simulink model "Q44444"  (R2016b)
settings: Solver=VariableStepAuto  StartTime=0.0  StopTime=100  RelTol=1e-3
values from neighbouring files (symbols this model uses):
  a0_const = 20    [Question_4.m]
  alpha = 0.3    [Question_4.m]
  p = 1000*eye(est_param)    [Question_4.m]
  t0 = B_prim_m    [Question_4.m]
  wn = sigma/zeta    [Question_4.m]
  zeta = ((log(Mp)^2)/(pi^2+log(Mp)^2))^0.5    [Question_4.m]
libraries: cstextras x2
settings Model: Creator=vaio  LastModifiedBy=user

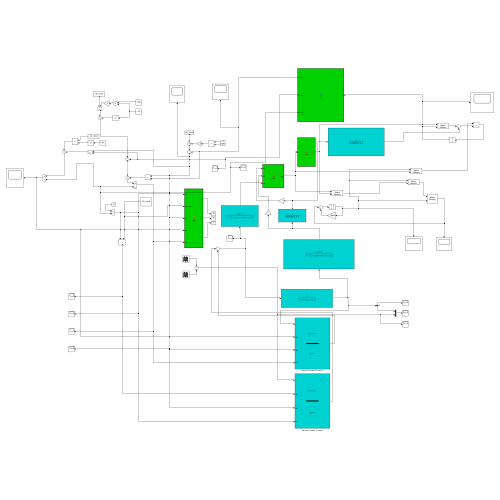
[thumbnail: Simulink's stored preview of the top-level diagram]
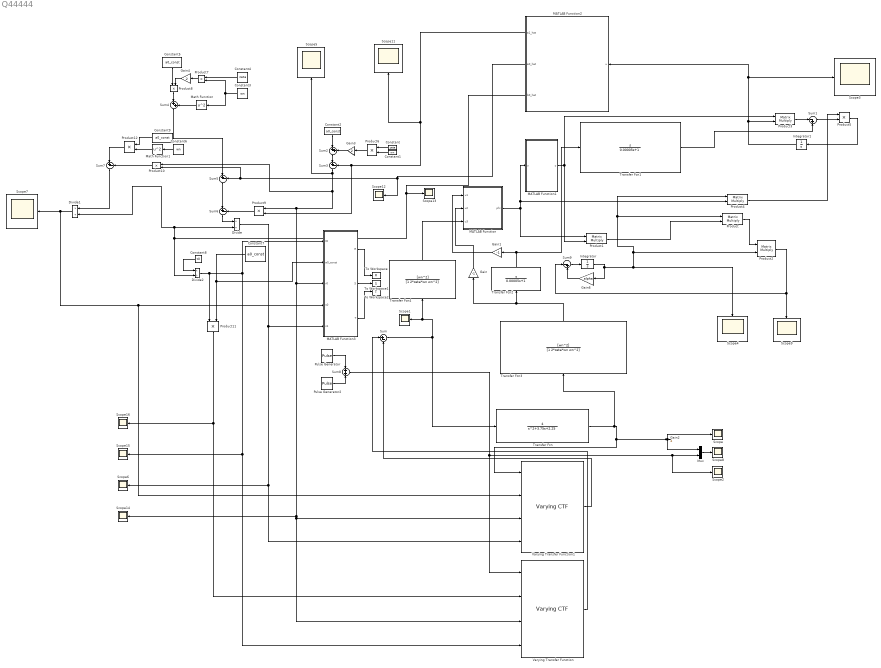
== system Q44444 ==
  Constant : Constant  Value=zeta
  Constant1 : Constant  Value=wn
  Constant{2,5,7,9} (4 alike) : Constant  Value=a0_const
  Constant3 : Constant  Value=wn
  Constant4 : Constant  Value=zeta
  Constant6 : Constant  Value=wn
  Constant8 : Constant  Value=t0
  Divide : Product  Inputs=*/
  Divide1 : Product  Inputs=*/
  Divide2 : Product  Inputs=*/
  Gain : Gain  Gain=-1
  Gain1 : Gain  Gain=-1
  Gain2 : Gain  Gain=4
  Gain3 : Gain  Gain=2
  Gain4 : Gain  Gain=2
  Gain6 : Gain  Gain=alpha
  Integrator : Integrator  InitialCondition=p  LimitOutput=on
  Integrator1 : Integrator  InitialCondition=[0.1;0.01;0.5]
  MATLAB Function : MATLAB Function  TreatAsAtomicUnit=on
  MATLAB Function1 : MATLAB Function  TreatAsAtomicUnit=on
  MATLAB Function2 : MATLAB Function  TreatAsAtomicUnit=on
  MATLAB Function3 : MATLAB Function  TreatAsAtomicUnit=on
  Math Function : Math  Operator=square  SaturateOnIntegerOverflow=on
  Math Function1 : Math  Operator=square  SaturateOnIntegerOverflow=on
  Mux : Mux  Inputs=2
  Product{,1..4} (5 alike) : Product  Multiplication=Matrix(*)
  Product{5..12} (8 alike) : Product
  Pulse Generator : DiscretePulseGenerator  PulseType=Time based  Amplitude=2  Period=50  PulseWidth=50
  Pulse Generator2 : DiscretePulseGenerator  PulseType=Time based  Amplitude=-2  Period=50  PulseWidth=50  PhaseDelay=25
  Scope{,1..9,11..16} (16 alike) : Scope
  Sum{,3,5..7} (5 alike) : Sum  Inputs=|+-
  Sum1 : Sum  Inputs=|-+
  Sum2 : Sum  Inputs=|++
  Sum4 : Sum  Inputs=|++
  Sum8 : Sum
  Sum9 : Sum  Inputs=|-+
  To Workspace : ToWorkspace  VariableName=R  SampleTime=-1
  To Workspace1 : ToWorkspace  VariableName=S  SampleTime=-1
  To Workspace2 : ToWorkspace  VariableName=T  SampleTime=-1
  Transfer Fcn : TransferFcn  Numerator=[4]  Denominator=[1 3.75 2.25]
  Transfer Fcn1 : TransferFcn  Numerator=[1 0]  Denominator=[0.00005 1]
  Transfer Fcn2 : TransferFcn  Numerator=[1 0]  Denominator=[0.00005 1]
  Transfer Fcn3 : TransferFcn  Numerator=[wn^2]  Denominator=[1 2*zeta*wn wn^2]
  Transfer Fcn4 : TransferFcn  Numerator=[wn^2]  Denominator=[1 2*zeta*wn wn^2]
  Varying Transfer Function : cstextras/Varying CTF  N=1
  Varying Transfer Function1 : cstextras/Varying CTF  N=1
  wires:
  Transfer Fcn2/1 -> Transfer Fcn1/1, Gain1/1
  Gain/1 -> MATLAB Function/2(u2)
  Sum/1 -> Transfer Fcn/1, Transfer Fcn4/1, Scope1/1
  Transfer Fcn3/1 -> Gain/1, Transfer Fcn2/1
  Integrator/1 -> Scope4/1, Product4/1, Product/1, Product2/2, Gain6/1
  Transfer Fcn4/1 -> MATLAB Function/3(u3)
  Gain1/1 -> MATLAB Function/1(u1)
  MATLAB Function/1(phi) -> Product4/2, MATLAB Function1/1(u), Product1/1
  MATLAB Function1/1(y) -> Product1/2, Product3/1
  Product1/1 -> Product/2
  Product/1 -> Product2/1
  Product2/1 -> Sum9/1, Scope9/1
  Integrator1/1 -> MATLAB Function2/1(u), Scope3/1, Product3/2
  Product3/1 -> Sum1/1
  Transfer Fcn1/1 -> Sum1/2
  Product4/1 -> Product5/1
  Sum1/1 -> Product5/2
  Product5/1 -> Integrator1/1
  Constant/1 -> Product6/1
  Constant1/1 -> Product6/2
  Product6/1 -> Gain3/1
  Gain3/1 -> Sum2/2
  Constant2/1 -> Sum2/1
  Sum2/1 -> Sum3/1
  MATLAB Function2/1(a1_hat) -> Sum3/2, Product9/2, Scope11/1
  Constant4/1 -> Product7/1
  Constant3/1 -> Math Function/1, Product7/2
  Product7/1 -> Gain4/1
  Gain4/1 -> Product8/2
  Constant5/1 -> Product8/1
  Math Function/1 -> Sum4/2
  Product8/1 -> Sum4/1
  Sum4/1 -> Sum5/1
  MATLAB Function2/2(a0_hat) -> Product10/2, Sum5/2, Scope12/1
  Sum5/1 -> Sum6/1
  Sum3/1 -> Product9/1, Varying Transfer Function1/3, Varying Transfer Function/3, Scope14/1, MATLAB Function3/3(r0), Product10/1, Scope5/1
  Product9/1 -> Sum6/2
  MATLAB Function2/3(b0_hat) -> Divide/2, Divide1/2, Divide2/2, Scope13/1
  Constant6/1 -> Math Function1/1
  Math Function1/1 -> Product12/2
  Product10/1 -> Sum7/2
  Sum7/1 -> Divide1/1
  Constant7/1 -> Product11/2, MATLAB Function3/2(a0_const)
  Constant8/1 -> Divide2/1
  Mux/1 -> Scope8/1
  Pulse Generator/1 -> Sum8/1
  Pulse Generator2/1 -> Sum8/2
  Sum8/1 -> Scope2/1, Mux/2, Varying Transfer Function/1
  Gain6/1 -> Sum9/2
  Sum9/1 -> Integrator/1
  Constant9/1 -> Product12/1
  Product12/1 -> Sum7/1
  MATLAB Function3/1(R) -> To Workspace/1
  MATLAB Function3/2(S) -> To Workspace1/1
  MATLAB Function3/3(T) -> To Workspace2/1
  Product11/1 -> Varying Transfer Function/2, Scope16/1
  Varying Transfer Function/1 -> Sum/1
  Transfer Fcn/1 -> Gain2/1, Varying Transfer Function1/1, Transfer Fcn3/1
  Varying Transfer Function1/1 -> Sum/2
  Divide2/1 -> Varying Transfer Function/4, Scope15/1, MATLAB Function3/1(t0), Product11/1
  Divide1/1 -> Varying Transfer Function1/2, MATLAB Function3/4(s0), Scope7/1
  Divide/1 -> Scope6/1, Varying Transfer Function1/4, MATLAB Function3/5(s1)
  Sum6/1 -> Divide/1
  Gain2/1 -> Scope/1, Mux/1

== matlab function Q44444/MATLAB Function1 ==
  data: u input; y output
function y = fcn(u)

y = u';

== matlab function Q44444/MATLAB Function ==
  data: u1 input; phi output; u2 input; u3 input
function phi = fcn(u1,u2,u3)
phi=[u1;u2;u3];

== matlab function Q44444/MATLAB Function2 ==
  data: u input; a1_hat output; a0_hat output; b0_hat output
function [a1_hat,a0_hat,b0_hat] = fcn(u)

a1_hat = u(1);
a0_hat=u(2);
b0_hat=u(3);

== matlab function Q44444/MATLAB Function3 ==
  data: t0 input; R output; S output; T output; a0_const input; r0 input; s0 input; s1 input
function [R,S,T] = fcn(t0,a0_const,r0,s0,s1)
% s=tf('s');
R =[1 r0];
S=[s0 s1];
T=[t0 t0*a0_const];
% R=1*s+r0;
% S=s0*s+s1;
% T=t0*s+t0*a0_const;
